simulink model "Subsystem"  (R2023b)
settings: Solver=FixedStepAuto  StartTime=0.0  StopTime=6  FixedStep=1  RelTol=1e-3
settings Model: Creator=alfre  LastModifiedBy=alfre
settings DataIOCC: SaveOutput=off  SaveTime=off

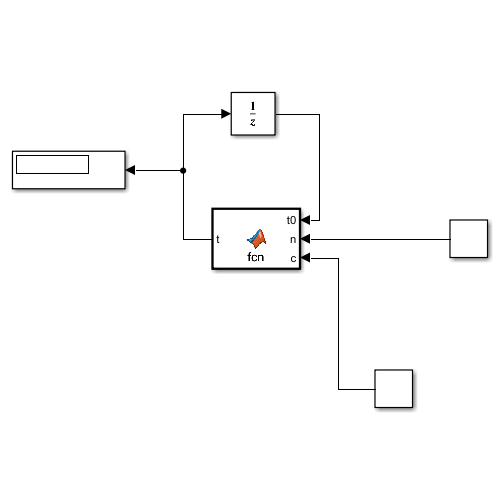
[thumbnail: Simulink's stored preview of the top-level diagram]
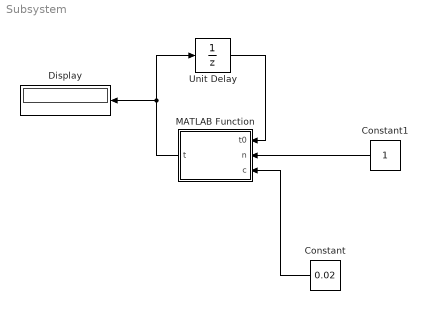
== system Subsystem ==
  Constant : Constant  Value=0.02
  Constant1 : Constant
  Display : Display
  MATLAB Function : MATLAB Function  TreatAsAtomicUnit=on
  Unit Delay : UnitDelay  InitialCondition=30  SampleTime=-1  HasFrameUpgradeWarning=on
  wires:
  Constant1/1 -> MATLAB Function/2(n)
  MATLAB Function/1(t) -> Unit Delay/1, Display/1
  Constant/1 -> MATLAB Function/3(c)
  Unit Delay/1 -> MATLAB Function/1(t0)

== matlab function Subsystem/MATLAB Function ==
  data: t0 input; t output; n input; c input
function t = fcn(t0, n, c)

t = t0 - n*c;
